simulink model "subsistema_carro"  (R2023b)
settings: Solver=VariableStepAuto  StartTime=0.0  StopTime=10.0  RelTol=1e-3
undefined symbols (not defined in the file): bt, btw, it, Jtd, Jtm_tb, Ktw, Mt, rtd
settings Model: Creator=nahue  LastModifiedBy=rodri

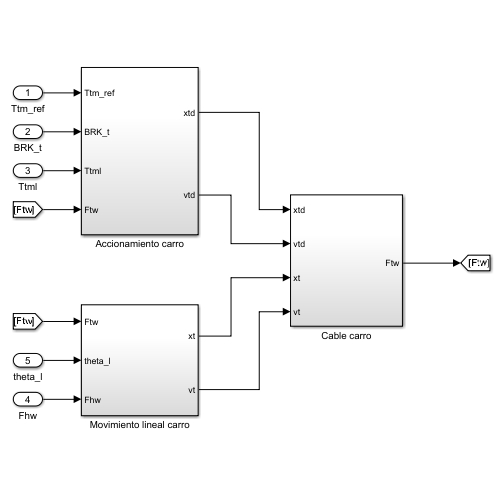
[thumbnail: Simulink's stored preview of the top-level diagram]
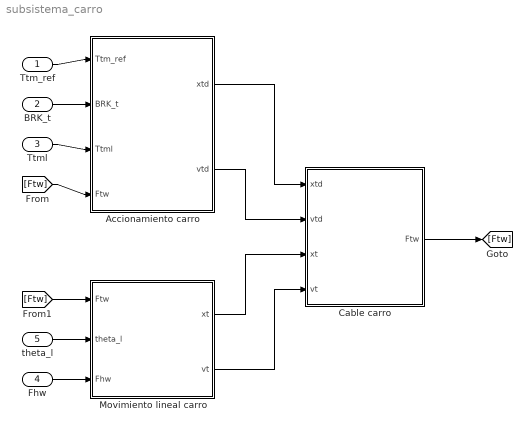
== system subsistema_carro ==
  Ttm_ref : Inport
  BRK_t : Inport  Port=2
  Ttml : Inport  Port=3
  Fhw : Inport  Port=4
  theta_l : Inport  Port=5
  Accionamiento carro : Subsystem
  Cable carro : Subsystem
  Movimiento lineal carro : Subsystem
  wires:
  Ttm_ref/1 -> Accionamiento carro/1(Ttm_ref)
  BRK_t/1 -> Accionamiento carro/2(BRK_t)
  Ttml/1 -> Accionamiento carro/3(Ttml)
  theta_l/1 -> Movimiento lineal carro/2(theta_l)
  Fhw/1 -> Movimiento lineal carro/3(Fhw)
  [Ftw] -> Accionamiento carro/4(Ftw)
  [Ftw] -> Movimiento lineal carro/1(Ftw)
  Accionamiento carro/1(xtd) -> Cable carro/1(xtd)
  Accionamiento carro/2(vtd) -> Cable carro/2(vtd)
  Movimiento lineal carro/1(xt) -> Cable carro/3(xt)
  Movimiento lineal carro/2(vt) -> Cable carro/4(vt)
  Cable carro/1(Ftw) -> [Ftw]

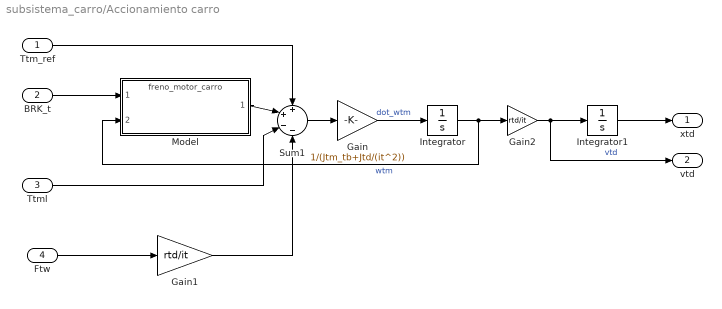
== system subsistema_carro/Accionamiento carro ==
  Ttm_ref : Inport
  BRK_t : Inport  Port=2
  Ttml : Inport  Port=3
  Ftw : Inport  Port=4
  Gain : Gain  Gain=1/(Jtm_tb+Jtd/(it^2))
  Gain1 : Gain  Gain=rtd/it
  Gain2 : Gain  Gain=rtd/it
  Integrator : Integrator
  Integrator1 : Integrator
  Model : ModelReference  ModelNameDialog=freno_motor_carro.slx  SimulationMode=Normal  ModelReferenceVersion=1.3
  Sum1 : Sum  Inputs=++--
  xtd : Outport
  vtd : Outport  Port=2
  wires:
  Model/1 -> Sum1/2
  Sum1/1 -> Gain/1
  Integrator/1 -> Gain2/1, Model/2  "wtm"
  Gain2/1 -> vtd/1, Integrator1/1  "vtd"
  Ttm_ref/1 -> Sum1/1
  Gain/1 -> Integrator/1  "dot_wtm"
  BRK_t/1 -> Model/1
  Integrator1/1 -> xtd/1
  Ttml/1 -> Sum1/3
  Ftw/1 -> Gain1/1
  Gain1/1 -> Sum1/4

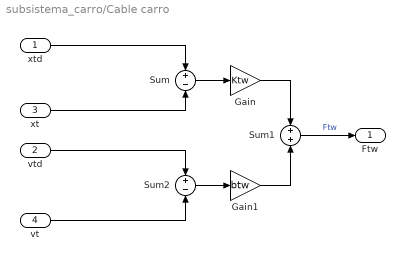
== system subsistema_carro/Cable carro ==
  xtd : Inport
  vtd : Inport  Port=2
  xt : Inport  Port=3
  vt : Inport  Port=4
  Gain : Gain  Gain=Ktw
  Gain1 : Gain  Gain=btw
  Sum : Sum  Inputs=+-
  Sum1 : Sum
  Sum2 : Sum  Inputs=+-
  Ftw : Outport
  wires:
  xtd/1 -> Sum/1
  Gain1/1 -> Sum1/2
  Sum/1 -> Gain/1
  xt/1 -> Sum/2
  Sum2/1 -> Gain1/1
  Gain/1 -> Sum1/1
  vt/1 -> Sum2/2
  Sum1/1 -> Ftw/1  "Ftw"
  vtd/1 -> Sum2/1

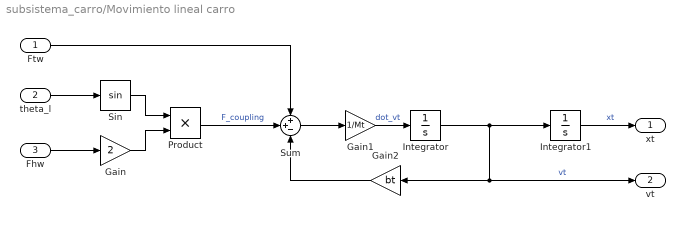
== system subsistema_carro/Movimiento lineal carro ==
  Ftw : Inport
  theta_l : Inport  Port=2
  Fhw : Inport  Port=3
  Gain : Gain  Gain=2
  Gain1 : Gain  Gain=1/Mt
  Gain2 : Gain  Gain=bt
  Integrator : Integrator
  Integrator1 : Integrator
  Product : Product
  Sin : Trigonometry
  Sum : Sum  Inputs=++-
  xt : Outport
  vt : Outport  Port=2
  wires:
  Gain1/1 -> Integrator/1  "dot_vt"
  Integrator/1 -> Gain2/1, vt/1, Integrator1/1  "vt"
  Gain2/1 -> Sum/3
  Sum/1 -> Gain1/1
  Integrator1/1 -> xt/1  "xt"
  Fhw/1 -> Gain/1
  Gain/1 -> Product/2
  theta_l/1 -> Sin/1
  Sin/1 -> Product/1
  Product/1 -> Sum/2  "F_coupling"
  Ftw/1 -> Sum/1
